simulink model "SWp4"  (R2016a)
settings: Solver=VariableStepAuto  StartTime=0.0  StopTime=10.0  RelTol=1e-3
libraries: simulink x2
settings Model: Creator=gdlau  LastModifiedBy=gdlau

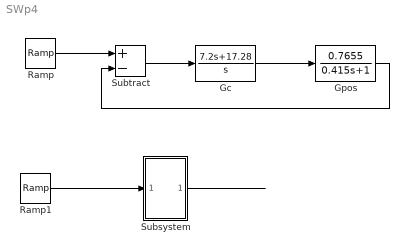
== system SWp4 ==
  Gc : TransferFcn  Numerator=[7.2 17.28]  Denominator=[1 0]
  Gpos : TransferFcn  Numerator=[0.7655]  Denominator=[0.415 1 ]
  Ramp : simulink/Sources/Ramp  slope=1  start=0  X0=0
  Ramp1 : simulink/Sources/Ramp  slope=1  start=0  X0=0
  Subsystem : Subsystem
  Subtract : Sum  Inputs=+-
  wires:
  Subtract/1 -> Gc/1
  Gc/1 -> Gpos/1
  Gpos/1 -> Subtract/2
  Ramp/1 -> Subtract/1
  Ramp1/1 -> Subsystem/1(In1)
  Subsystem/1(Out1) -> ?

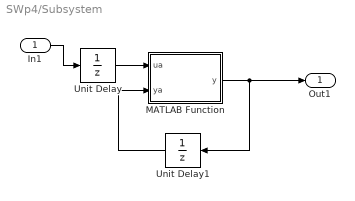
== system SWp4/Subsystem ==
  In1 : Inport
  MATLAB Function : MATLAB Function  TreatAsAtomicUnit=on
  Unit Delay : UnitDelay  SampleTime=-1
  Unit Delay1 : UnitDelay  SampleTime=-1
  Out1 : Outport
  wires:
  In1/1 -> Unit Delay/1
  Unit Delay/1 -> MATLAB Function/1(ua)
  MATLAB Function/1(y) -> Out1/1, Unit Delay1/1
  Unit Delay1/1 -> MATLAB Function/2(ya)

== matlab function SWp4/Subsystem/MATLAB Function ==
  data: ua input; y output; ya input
function y = ControladorP4(ua, ya)
%#codegen
a = 1.008
b = 0.0817
c = 0.07353
d = 3.647*10^(-7) 
y = a*ua + b*ua + c*ya - d*ya;
